simulink model "APP_Sensor1_2"  (R2021a)
settings: Solver=VariableStepAuto  StartTime=0.0  StopTime=10.0  RelTol=1e-3
libraries: simulink x2
settings Model: Creator=lenovo  LastModifiedBy=lenovo

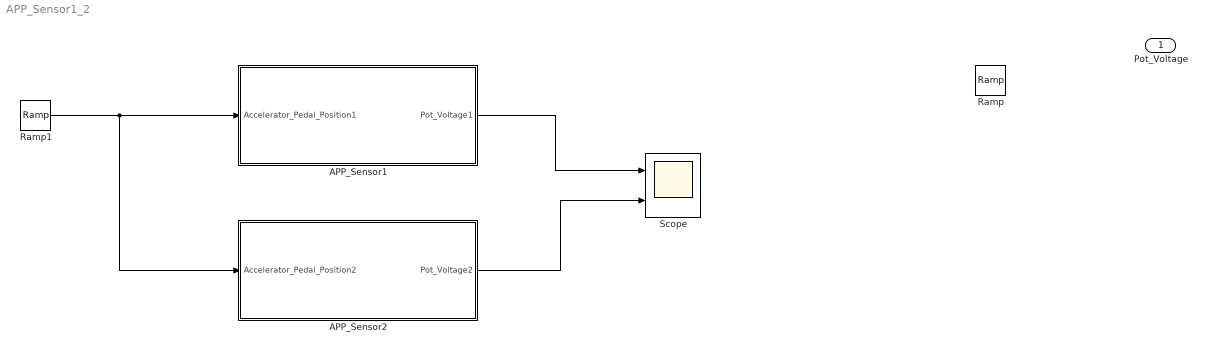
== system APP_Sensor1_2 ==
  APP_Sensor1 : Subsystem
  APP_Sensor2 : Subsystem
  Ramp : simulink/Sources/Ramp  slope=1  start=0  InitialOutput=0
  Ramp1 : simulink/Sources/Ramp  slope=4  start=0  InitialOutput=0.5
  Scope : Scope  NumInputPorts=2
  Pot_Voltage : Outport
  wires:
  Ramp1/1 -> APP_Sensor2/1(Accelerator_Pedal_Position2), APP_Sensor1/1(Accelerator_Pedal_Position1)
  APP_Sensor1/1(Pot_Voltage1) -> Scope/1
  APP_Sensor2/1(Pot_Voltage2) -> Scope/2

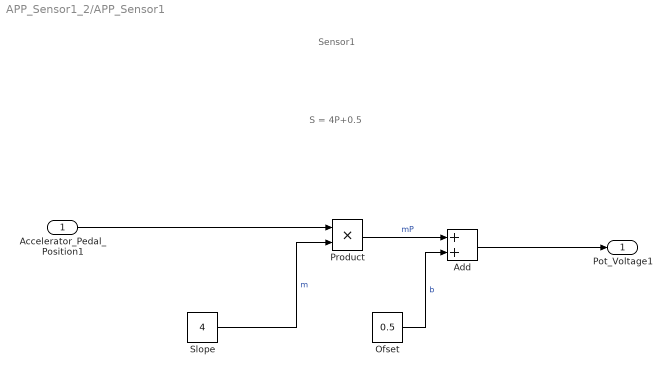
== system APP_Sensor1_2/APP_Sensor1 ==
  note: S = 4P+0.5
  note: Sensor1
  Accelerator_Pedal_Position1 : Inport
  Add : Sum
  Ofset : Constant  Value=0.5
  Product : Product
  Slope : Constant  Value=4
  Pot_Voltage1 : Outport
  wires:
  Slope/1 -> Product/2  "m"
  Ofset/1 -> Add/2  "b"
  Product/1 -> Add/1  "mP"
  Accelerator_Pedal_Position1/1 -> Product/1
  Add/1 -> Pot_Voltage1/1

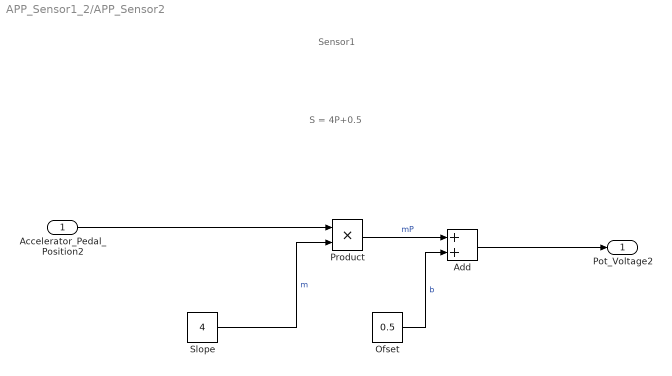
== system APP_Sensor1_2/APP_Sensor2 ==
  note: Sensor1
  note: S = 4P+0.5
  Accelerator_Pedal_Position2 : Inport
  Add : Sum
  Ofset : Constant  Value=0.5
  Product : Product
  Slope : Constant  Value=4
  Pot_Voltage2 : Outport
  wires:
  Add/1 -> Pot_Voltage2/1
  Accelerator_Pedal_Position2/1 -> Product/1
  Product/1 -> Add/1  "mP"
  Ofset/1 -> Add/2  "b"
  Slope/1 -> Product/2  "m"
